simulink model "stabilization2311"  (R2024a)
settings: Solver=VariableStepAuto  StartTime=0.0  StopTime=10  RelTol=1e-3
settings Model: Creator=pupkinzalupkin  LastModifiedBy=pupkinzalupkin

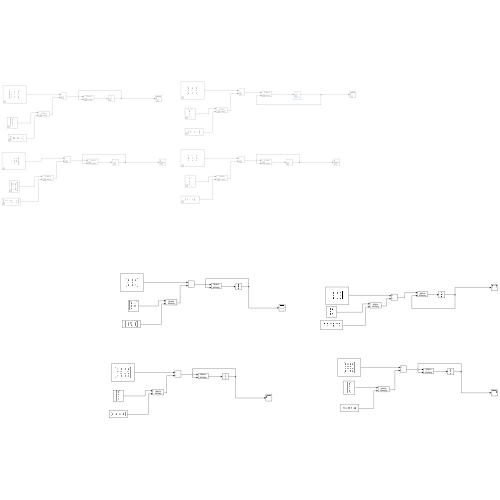
[thumbnail: Simulink's stored preview of the top-level diagram]
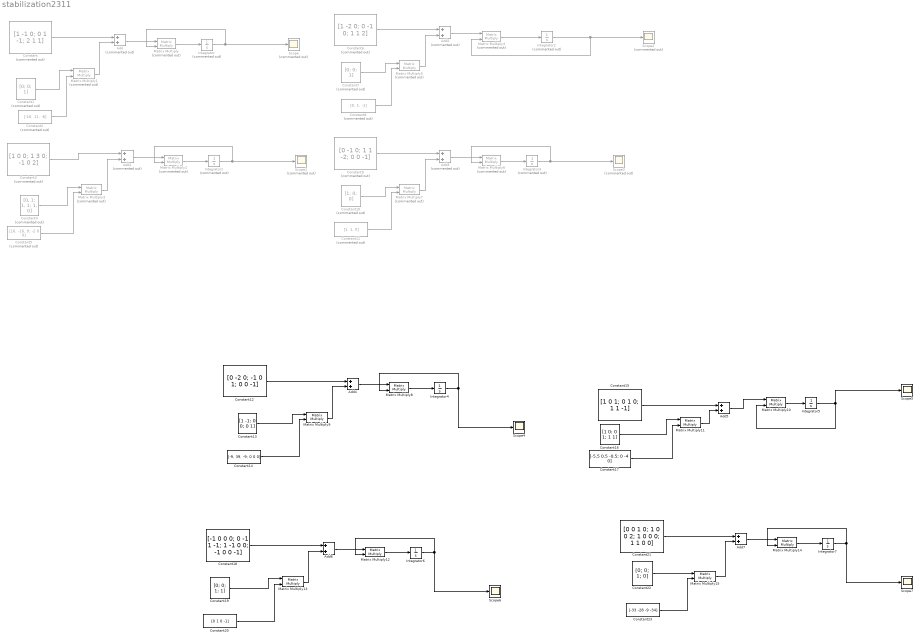
== system stabilization2311 ==
  Add{,1..3} (4 alike) : Sum  Commented=on
  Add{4..7} (4 alike) : Sum
  Constant : Constant  Commented=on  Value=[1 -1 0; 0 1 -1; 2 1 1]
  Constant1 : Constant  Commented=on  Value=[0; 0; 1]  VectorParams1D=off
  Constant10 : Constant  Commented=on  Value=[1; 0; 0]  VectorParams1D=off
  Constant11 : Constant  Commented=on  Value=[1, 1, 0]  VectorParams1D=off
  Constant12 : Constant  Value=[0 -2 0; -1 0 1; 0 0 -1]
  Constant13 : Constant  Value=[1 -1; 0 0; 0 1]  VectorParams1D=off
  Constant14 : Constant  Value=[-9, 39, -9; 0 0 0]  VectorParams1D=off
  Constant15 : Constant  Value=[1 0 1; 0 1 0; 1 1 -1]
  Constant16 : Constant  Value=[1 0; 0 1; 1 1]  VectorParams1D=off
  Constant17 : Constant  Value=[-5.5 0.5 -0.5; 0 -4 0]  VectorParams1D=off
  Constant18 : Constant  Value=[-1 0 0 0; 0 -1 1 -1; 1 -1 0 0; -1 0 0 -1]
  Constant19 : Constant  Value=[0; 0; 1; 1]  VectorParams1D=off
  Constant2 : Constant  Commented=on  Value=[-10, 11, -6]  VectorParams1D=off
  Constant20 : Constant  Value=[0 1 0 -1]  VectorParams1D=off
  Constant21 : Constant  Value=[0 0 1 0; 1 0 0 2; 1 0 0 0; 1 1 0 0]
  Constant22 : Constant  Value=[0; 0; 1; 0]  VectorParams1D=off
  Constant23 : Constant  Value=[-33 -28 -9 -34]  VectorParams1D=off
  Constant3 : Constant  Commented=on  Value=[1 0 0; 1 3 0; -1 0 2]
  Constant4 : Constant  Commented=on  Value=[0, 1; 1, 1; 1, 0]  VectorParams1D=off
  Constant5 : Constant  Commented=on  Value="[16,  -16, 9; -2 0 0]"  VectorParams1D=off
  Constant6 : Constant  Commented=on  Value=[1 -2 0; 0 -1 0; 1 1 2]
  Constant7 : Constant  Commented=on  Value=[0; 0; 1]  VectorParams1D=off
  Constant8 : Constant  Commented=on  Value=[0, 1, -1]  VectorParams1D=off
  Constant9 : Constant  Commented=on  Value=[0 -1 0; 1 1 -2; 0 0 -1]
  Integrator{,1..3} (4 alike) : Integrator  Commented=on  InitialCondition=[0; 0; -1]
  Integrator4 : Integrator  InitialCondition=[0; 0; -1]
  Integrator5 : Integrator  InitialCondition=[0; 1; 0]
  Integrator6 : Integrator  InitialCondition=[0; 0; -1; -1]
  Integrator7 : Integrator  InitialCondition=[0; 0; 0; -1]
  Matrix Multiply{,1..7} (8 alike) : Product  Commented=on  Multiplication=Matrix(*)
  Matrix Multiply{8..15} (8 alike) : Product  Multiplication=Matrix(*)
  Scope{,1..3} (4 alike) : Scope  Commented=on
  Scope{4..7} (4 alike) : Scope
  wires:
  Matrix Multiply/1 -> Integrator/1
  Integrator/1 -> Matrix Multiply/2, Scope/1
  Constant/1 -> Add/1
  Add/1 -> Matrix Multiply/1
  Constant1/1 -> Matrix Multiply1/1
  Constant2/1 -> Matrix Multiply1/2
  Matrix Multiply1/1 -> Add/2
  Matrix Multiply3/1 -> Add1/2
  Constant5/1 -> Matrix Multiply3/2
  Matrix Multiply2/1 -> Integrator1/1
  Add1/1 -> Matrix Multiply2/1
  Integrator1/1 -> Matrix Multiply2/2, Scope1/1
  Constant4/1 -> Matrix Multiply3/1
  Constant3/1 -> Add1/1
  Matrix Multiply5/1 -> Add2/2
  Constant8/1 -> Matrix Multiply5/2
  Matrix Multiply4/1 -> Integrator2/1
  Add2/1 -> Matrix Multiply4/1
  Integrator2/1 -> Scope2/1, Matrix Multiply4/2
  Constant7/1 -> Matrix Multiply5/1
  Constant6/1 -> Add2/1
  Constant11/1 -> Matrix Multiply7/2
  Matrix Multiply6/1 -> Integrator3/1
  Constant10/1 -> Matrix Multiply7/1
  Constant9/1 -> Add3/1
  Integrator3/1 -> Matrix Multiply6/2, Scope3/1
  Add3/1 -> Matrix Multiply6/1
  Matrix Multiply7/1 -> Add3/2
  Constant14/1 -> Matrix Multiply9/2
  Matrix Multiply8/1 -> Integrator4/1
  Matrix Multiply9/1 -> Add4/2
  Add4/1 -> Matrix Multiply8/1
  Integrator4/1 -> Matrix Multiply8/2, Scope4/1
  Constant13/1 -> Matrix Multiply9/1
  Constant12/1 -> Add4/1
  Matrix Multiply10/1 -> Integrator5/1
  Constant15/1 -> Add5/1
  Matrix Multiply11/1 -> Add5/2
  Add5/1 -> Matrix Multiply10/1
  Constant17/1 -> Matrix Multiply11/2
  Integrator5/1 -> Scope5/1, Matrix Multiply10/2
  Constant16/1 -> Matrix Multiply11/1
  Matrix Multiply12/1 -> Integrator6/1
  Constant18/1 -> Add6/1
  Matrix Multiply13/1 -> Add6/2
  Add6/1 -> Matrix Multiply12/1
  Constant20/1 -> Matrix Multiply13/2
  Integrator6/1 -> Matrix Multiply12/2, Scope6/1
  Constant19/1 -> Matrix Multiply13/1
  Matrix Multiply14/1 -> Integrator7/1
  Constant22/1 -> Matrix Multiply15/1
  Constant21/1 -> Add7/1
  Matrix Multiply15/1 -> Add7/2
  Constant23/1 -> Matrix Multiply15/2
  Integrator7/1 -> Matrix Multiply14/2, Scope7/1
  Add7/1 -> Matrix Multiply14/1
